simulink model "RL_PID_pruebasHIL"  (R2022b)
settings: Solver=FixedStepAuto  StartTime=0.0  StopTime=10.0  RelTol=1e-3
InitFcn:
  | m=200;
  | g=9.81;
  | suelo = 0.0225;
  | techo = 0.01;
  | lev_nom = 0.01965;
  | time_stp = 2;
  | load('hems.mat');
undefined symbols (not defined in the file): hems
settings Model: Creator=aceao  LastModifiedBy=aceao
settings OptimizationCC: DefaultParameterBehavior=Inlined  UseDivisionForNetSlopeComputation=on  GainParamInheritBuiltInType=on  UseFloatMulNetSlope=on  InlineInvariantSignals=on  PassReuseOutputArgsAs=Individual arguments  ZeroExternalMemoryAtStartup=off  ZeroInternalMemoryAtStartup=off  NoFixptDivByZeroProtection=on  EfficientFloat2IntCast=on  LifeSpan=1  OptimizeBlockOrder=speed  DifferentSizesBufferReuse=on  EfficientTunableParamExpr=on
settings DebuggingCC: ParameterTunabilityLossMsg=error
settings HardwareCC: ProdBitPerPointer=32  ProdBitPerSizeT=32  ProdBitPerPtrDiffT=32  ProdLargestAtomicFloat=None  ProdWordSize=32  ProdLongLongMode=on  ProdHWDeviceType=Custom Processor->Custom Processor
settings SFSimCC: MATLABDynamicMemAlloc=off
settings RTWCC: Description=Embedded Coder  SystemTargetFile=ert.tlc  TemplateMakefile=ert_default_tmf
settings CodeAppCC: ForceParamTrailComments=on  IgnoreCustomStorageClasses=off  OperatorAnnotations=on  SimulinkDataObjDesc=on  SFDataObjDesc=on  CustomSymbolStrGlobalVar=rt$N$M  CustomSymbolStrType=$N$M  CustomSymbolStrFcn=$N$M$F  CustomSymbolStrMacro=$N$M  InsertBlockDesc=on
settings ERTTargetCC: TargetLangStandard=C99 (ISO)  GenerateSampleERTMain=on  IncludeMdlTerminateFcn=off  CombineSignalStateStructs=on  SupportComplex=off  SupportContinuousTime=on  InlinedParameterPlacement=NonHierarchical  ERTCustomFileTemplate=example_file_process.tlc  ERTFilePackagingFormat=CompactWithDataFile

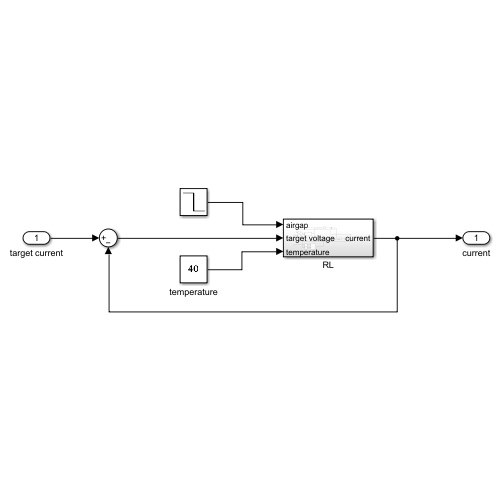
[thumbnail: Simulink's stored preview of the top-level diagram]
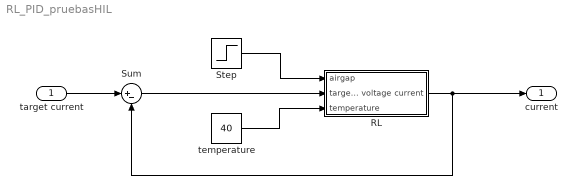
== system RL_PID_pruebasHIL ==
  target current : Inport
  RL : Subsystem
  Step : Step  Before=suelo  After=lev_nom  SampleTime=0
  Sum : Sum  Inputs=|+-
  temperature : Constant  Value=40
  current : Outport
  wires:
  temperature/1 -> RL/3(temperature)
  target current/1 -> Sum/1
  Sum/1 -> RL/2(target voltage)
  RL/1(current) -> Sum/2, current/1
  Step/1 -> RL/1(airgap)

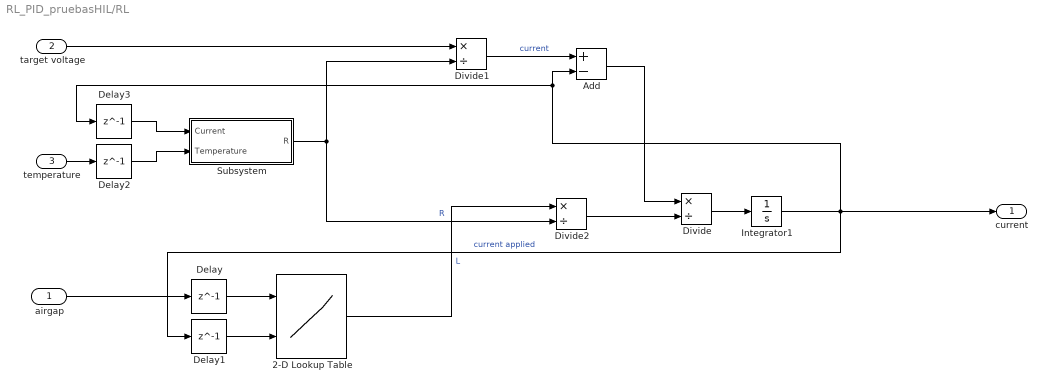
== system RL_PID_pruebasHIL/RL ==
  airgap : Inport
  target voltage : Inport  Port=2
  temperature : Inport  Port=3
  2-D Lookup Table : Lookup_n-D  BreakpointsForDimension1=hems.Airgap  BreakpointsForDimension2=hems.Current(2:110)  Table=hems.Inductance  InternalRulePriority=Speed  RndMeth=Simplest
      settings: InputPortMap=u0,u1
  Add : Sum  Inputs=+-
  Delay{,1..3} (4 alike) : Delay  DelayLength=1
  Divide : Product  Inputs=*/
  Divide1 : Product  Inputs=*/
  Divide2 : Product  Inputs=*/
  Integrator1 : Integrator
  Subsystem : Subsystem
  current : Outport
  wires:
  2-D Lookup Table/1 -> Divide2/1  "L"
  Integrator1/1 -> Delay1/1, current/1, Delay3/1, Add/2  "current applied"
  Delay1/1 -> 2-D Lookup Table/2
  Delay3/1 -> Subsystem/1(Current)
  Delay/1 -> 2-D Lookup Table/1
  Subsystem/1(R) -> Divide2/2, Divide1/2  "R"
  Divide2/1 -> Divide/2
  Delay2/1 -> Subsystem/2(Temperature)
  airgap/1 -> Delay/1
  Divide1/1 -> Add/1  "current"
  target voltage/1 -> Divide1/1
  Add/1 -> Divide/1
  Divide/1 -> Integrator1/1
  temperature/1 -> Delay2/1

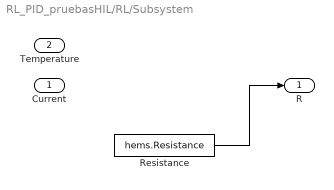
== system RL_PID_pruebasHIL/RL/Subsystem ==
  Current : Inport
  Temperature : Inport  Port=2
  Resistance : Constant  Value=hems.Resistance
  R : Outport
  wires:
  Resistance/1 -> R/1
